simulink model "QAM_HF_Modell_Beispiel1"  (R2025b)
settings: Solver=VariableStepAuto  StartTime=0.0  StopTime=10.0  RelTol=1e-3
values from neighbouring files (symbols this model uses):
  ADC_delta = (ADC_Vmax - ADC_Vmin) / ADC_levels    (= 0.001953125)    [QAM_Bewertung_System_Parameter.m]
  alpha_LG = 0.001    [QAM_Bewertung_System_Parameter.m]
  c_init = complex(zeros(N_coef,1))    [QAM_Bewertung_System_Parameter.m]
  DAC_delta = (DAC_Vmax - DAC_Vmin) / DAC_levels    (= 0.000244140625)    [QAM_Bewertung_System_Parameter.m]
  freq_offset_Hz = 50    [QAM_Bewertung_System_Parameter.m]
  Fs = Rs * sps    (= 358400000)    [QAM_Bewertung_System_Parameter.m]
  Gain_DAC = V_dac_rms / sqrt(TX_Power)    [QAM_Bewertung_System_Parameter.m]
  Gain_rx_dB = 20*log10(Gain_rx_linear)    [QAM_Bewertung_System_Parameter.m]
  Gain_Tx_dB = 24    [QAM_Bewertung_System_Parameter.m]
  gainI_RX_dB = 0    [QAM_Bewertung_System_Parameter.m]
  gainI_TX_dB = 0.5    [QAM_Bewertung_System_Parameter.m]
  gainQ_RX_dB = 0.5    [QAM_Bewertung_System_Parameter.m]
  gainQ_TX_dB = 0.5    [QAM_Bewertung_System_Parameter.m]
  K_LG = 0.02    [QAM_Bewertung_System_Parameter.m]
  L_total_dB = FSPL_dB + L_gas_dB + L_rain_dB + L_sys_dB    [QAM_Bewertung_System_Parameter.m]
  LO_leakage_RX_dB = -30    [QAM_Bewertung_System_Parameter.m]
  LO_leakage_TX_dB = -35    [QAM_Bewertung_System_Parameter.m]
  M = 256    [QAM_Bewertung_System_Parameter.m]
  Memory = 1    [QAM_Bewertung_System_Parameter.m]
  mu = 5e-4    (= 0.0005)    [QAM_Bewertung_System_Parameter.m]
  mu_DPD = 1e-5    (= 1e-05)    [QAM_Bewertung_System_Parameter.m]
  numOrders = 3    [QAM_Bewertung_System_Parameter.m]
  P1dB_dBm = 20    [QAM_Bewertung_System_Parameter.m]
  P_TX_dBm = 10*log10(P_TX_W*1e3)    [QAM_Bewertung_System_Parameter.m]
  P_TX_W = 2    [QAM_Bewertung_System_Parameter.m]
  PAPR_dB = 6    [QAM_Bewertung_System_Parameter.m]
  phaseMismatch_RX_deg = 1    [QAM_Bewertung_System_Parameter.m]
  phaseMismatch_TX_deg = 1    [QAM_Bewertung_System_Parameter.m]
  PN_RX_std_deg = 0.01    [QAM_Bewertung_System_Parameter.m]
  PN_TX_std_deg = 0.01    [QAM_Bewertung_System_Parameter.m]
  R = 50    [QAM_Bewertung_System_Parameter.m]
  simulink_params = struct()    [QAM_Bewertung_System_Parameter.m]
  Z0 = 50    [QAM_Bewertung_System_Parameter.m]
libraries: dspstat3 x8, simulink_extras x4, dspmathops x3, simulink x2, commsink2 x2, commfilt2 x2, commdigbbndam3 x2, commrfcorlib x1, rfmathmodels2 x1, commrandsrc3 x1
settings Model: Creator=giand  LastModifiedBy=giand

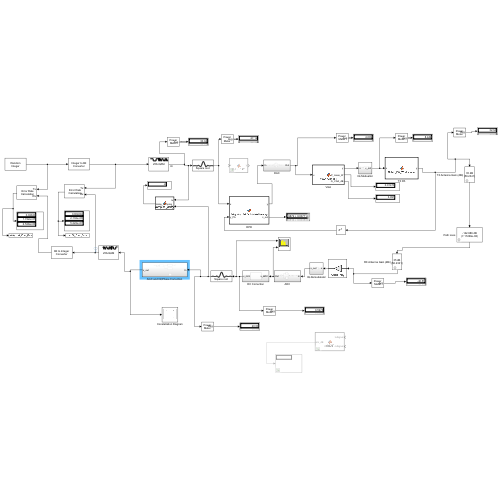
[thumbnail: Simulink's stored preview of the top-level diagram]
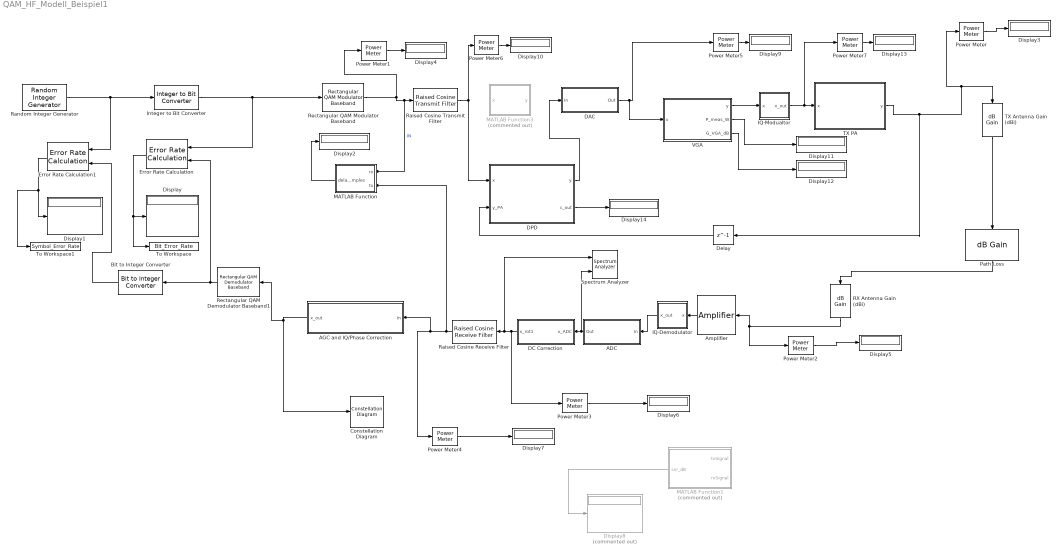
== system QAM_HF_Modell_Beispiel1 ==
  ADC : Subsystem
  AGC and IQ/Phase Correction : Subsystem
  Amplifier : rfmathmodels2/Amplifier  Model=cubic  Gain=Gain_rx_dB  Nonlinearity=OIP3  IIP3=Inf  OIP3=Inf  IP1dB=Inf  OP1dB=Inf  IPsat=Inf  OPsat=Inf  Table=[ -25, 5, -1; -10, 20, -2; 0, 27, 5; 5, 28, 12 ]  MagnitudeGainDB=0  Vsat=1  MagnitudeSmooth=2  PhaseGainRadian=-.45  PhaseSaturation=.88  PhaseSmooth=[ 3.43, 3.43 ]  InputScaleDB=0  AmAmParameters=[ 2.1587, 1.1517 ]  AmPmParameters=[ 4.0033, 9.1040 ]  OutputScaleDB=0  SimulateUsing=Interpreted execution  IncludeNoise=on  NoiseType=NF  NoiseTemperature=290  NF=NF_required_dB  NoiseFactor=2  SeedSource=auto  Seed=67987  SampleRate=1e6
  Bit to Integer Converter : simulink/Logic and Bit Operations/Bit to Integer Converter  nbits=k  bitOrder=MSB first  signedOutputValues=Unsigned  outDtype=Inherit via internal rule  outDtypeSigned=Inherit via internal rule
  Constellation Diagram : ConstellationDiagram  WindowPosition=[606.000000,-23.000000,853.000000,842.000000,]  Visible=on  ScopeFrameLocation=window
  DAC : Subsystem
  DC Correction : Subsystem
  DPD : MATLAB Function  TreatAsAtomicUnit=on
  Delay : Delay  DelayLength=1  InitialCondition=0
  Display{,1..7,9..14} (14 alike) : Display
  Display8 : Display  Commented=on
  Error Rate Calculation : commsink2/Error Rate Calculation  N=simulink_params.rrc_span*log2(M)  st_delay=0  cp_mode=Entire frame  subframe=[]  PMode=Port  WsName=ErrorVec  RsMode2=off  stop=off  numErr=100  maxBits=1e6
  Error Rate Calculation1 : commsink2/Error Rate Calculation  N=simulink_params.rrc_span  st_delay=0  cp_mode=Entire frame  subframe=[]  PMode=Port  WsName=ErrorVec  RsMode2=off  stop=off  numErr=100  maxBits=1e6
  IQ-Demodulator : Subsystem
  IQ-Modualtor : Subsystem
  Integer to Bit Converter : simulink/Logic and Bit Operations/Integer to Bit Converter  nbits=simulink_params.k  signedInputValues=Unsigned  bitOrder=MSB first  outDtype=Inherit via internal rule
      settings: LibrarySourceBlock=|
      | commutil2/Integer to Bit
      | Converter
  MATLAB Function : MATLAB Function  TreatAsAtomicUnit=on
  MATLAB Function1 : MATLAB Function  Commented=on  TreatAsAtomicUnit=on
  MATLAB Function3 : MATLAB Function  Commented=on  TreatAsAtomicUnit=on
  Path Loss : dspmathops/dB Gain  dB=-L_total_dB  intype=Amplitude
  Power Meter : dspstat3/Power Meter  Measurement=Average power  ReferenceLoad=R  OutputPowerUnits=dBm  WindowLength=256  OverlapLength=255  AllowArbitraryInputLength=off  ComputeCCDF=off  PowerRange=50  PowerResolution=0.1  CCDFOutput=Relative power (dB above average power)  ProbabilityVector=[ 10; 1; 0.1; 0.01; 0.001; 0.0001 ]  RelativePowerVector=[ 0; 3; 6; 9; 12 ]  ResetPort=off  SimulateUsing=Code generation
      settings: LibrarySourceBlock=commutil2/Power Meter
  Power Meter1 : dspstat3/Power Meter  Measurement=Average power  ReferenceLoad=1  OutputPowerUnits=dBm  WindowLength=256  OverlapLength=255  AllowArbitraryInputLength=on  ComputeCCDF=off  PowerRange=50  PowerResolution=0.1  CCDFOutput=Relative power (dB above average power)  ProbabilityVector=[ 10; 1; 0.1; 0.01; 0.001; 0.0001 ]  RelativePowerVector=[ 0; 3; 6; 9; 12 ]  ResetPort=off  SimulateUsing=Code generation
      settings: LibrarySourceBlock=commutil2/Power Meter
  Power Meter2 : dspstat3/Power Meter  Measurement=Average power  ReferenceLoad=R  OutputPowerUnits=dBm  WindowLength=256  OverlapLength=255  AllowArbitraryInputLength=off  ComputeCCDF=off  PowerRange=50  PowerResolution=0.1  CCDFOutput=Relative power (dB above average power)  ProbabilityVector=[ 10; 1; 0.1; 0.01; 0.001; 0.0001 ]  RelativePowerVector=[ 0; 3; 6; 9; 12 ]  ResetPort=off  SimulateUsing=Code generation
      settings: LibrarySourceBlock=commutil2/Power Meter
  Power Meter3 : dspstat3/Power Meter  Measurement=Average power  ReferenceLoad=R  OutputPowerUnits=dBm  WindowLength=256  OverlapLength=255  AllowArbitraryInputLength=off  ComputeCCDF=off  PowerRange=50  PowerResolution=0.1  CCDFOutput=Relative power (dB above average power)  ProbabilityVector=[ 10; 1; 0.1; 0.01; 0.001; 0.0001 ]  RelativePowerVector=[ 0; 3; 6; 9; 12 ]  ResetPort=off  SimulateUsing=Code generation
      settings: LibrarySourceBlock=commutil2/Power Meter
  Power Meter4 : dspstat3/Power Meter  Measurement=Average power  ReferenceLoad=1  OutputPowerUnits=dBm  WindowLength=256  OverlapLength=255  AllowArbitraryInputLength=off  ComputeCCDF=off  PowerRange=50  PowerResolution=0.1  CCDFOutput=Relative power (dB above average power)  ProbabilityVector=[ 10; 1; 0.1; 0.01; 0.001; 0.0001 ]  RelativePowerVector=[ 0; 3; 6; 9; 12 ]  ResetPort=off  SimulateUsing=Code generation
      settings: LibrarySourceBlock=commutil2/Power Meter
  Power Meter5 : dspstat3/Power Meter  Measurement=Average power  ReferenceLoad=R  OutputPowerUnits=dBm  WindowLength=256  OverlapLength=255  AllowArbitraryInputLength=on  ComputeCCDF=off  PowerRange=50  PowerResolution=0.1  CCDFOutput=Relative power (dB above average power)  ProbabilityVector=[ 10; 1; 0.1; 0.01; 0.001; 0.0001 ]  RelativePowerVector=[ 0; 3; 6; 9; 12 ]  ResetPort=off  SimulateUsing=Code generation
      settings: LibrarySourceBlock=commutil2/Power Meter
  Power Meter6 : dspstat3/Power Meter  Measurement=Average power  ReferenceLoad=1  OutputPowerUnits=dBm  WindowLength=256  OverlapLength=255  AllowArbitraryInputLength=on  ComputeCCDF=off  PowerRange=50  PowerResolution=0.1  CCDFOutput=Relative power (dB above average power)  ProbabilityVector=[ 10; 1; 0.1; 0.01; 0.001; 0.0001 ]  RelativePowerVector=[ 0; 3; 6; 9; 12 ]  ResetPort=off  SimulateUsing=Code generation
      settings: LibrarySourceBlock=commutil2/Power Meter
  Power Meter7 : dspstat3/Power Meter  Measurement=Average power  ReferenceLoad=R  OutputPowerUnits=dBm  WindowLength=256  OverlapLength=255  AllowArbitraryInputLength=on  ComputeCCDF=off  PowerRange=50  PowerResolution=0.1  CCDFOutput=Relative power (dB above average power)  ProbabilityVector=[ 10; 1; 0.1; 0.01; 0.001; 0.0001 ]  RelativePowerVector=[ 0; 3; 6; 9; 12 ]  ResetPort=off  SimulateUsing=Code generation
      settings: LibrarySourceBlock=commutil2/Power Meter
  RX Antenna Gain (dBi) : dspmathops/dB Gain  dB=G_TX_dBi  intype=Amplitude
  Raised Cosine Receive Filter : commfilt2/Raised Cosine Receive Filter  filtType=Square root  R=simulink_params.rrc_rolloff  filtSpan=simulink_params.rrc_span  N=simulink_params.sps  downFactor=simulink_params.sps  downOffset=0  filterGain=1  InputProcessing=Columns as channels (frame based)  RateOptions=Enforce single-rate processing  framing=Mute  checkCoeff=off  variableName=rcRxFilt  currentFiltSpan=10  D=5  inputOffset=0  sampMode=Mute  saveAsFlag=0  rateMode=Downsampling  checkGain=Normalized  launchFVT=on  roundingMode=Floor  overflowMode=off  coeffDataTypeStr=Inherit: Same word length as input  coeffMin=[]  coeffMax=[]  coeffLastDataTypeStr=Inherit: Same word length as input  accumDataTypeStr=Inherit: Same as product output  accumLastDataTypeStr=Inherit: Same as product output  outputDataTypeStr=Inherit: Same as accumulator  outputMin=[]  outputMax=[]  outputLastDataTypeStr=Inherit: Same as accumulator
  Raised Cosine Transmit Filter : commfilt2/Raised Cosine Transmit Filter  filtType=Square root  R=simulink_params.rrc_rolloff  filtSpan=simulink_params.rrc_span  N=simulink_params.sps  filterGain=1  InputProcessing=Columns as channels (frame based)  RateOptions=Enforce single-rate processing  framing=Mute  checkCoeff=off  variableName=rcTxFilt  checkGain=Normalized  sampMode=Mute  saveAsFlag=0  currentFiltSpan=10  D=(10)/2  launchFVT=on  roundingMode=Floor  overflowMode=off  coeffDataTypeStr=Inherit: Same word length as input  coeffMin=[]  coeffMax=[]  coeffLastDataTypeStr=Inherit: Same word length as input  outputDataTypeStr=Inherit: Same as accumulator  outputMin=[]  outputMax=[]  outputLastDataTypeStr=Inherit: Same as accumulator
  Random Integer Generator : commrandsrc3/Random Integer Generator  SetSize=simulink_params.M  SeedSource=Auto  Seed=0  SampleTime=1/simulink_params.Rs  SamplesPerFrame=simulink_params.spf  OutputDataType=double  SimulateUsing=Interpreted execution
  Rectangular QAM Demodulator Baseband1 : commdigbbndam3/Rectangular QAM Demodulator Baseband  M=M  OutType=Bit  DecType=Hard decision  VarSource=Dialog  Variance=1  Dec=Gray  Mapping=[0:15]  PowType=Average Power  MinDist=2  AvgPow=1  PeakPow=1  Ph=0  outDtype1=Inherit via internal rule  outDtype2=Inherit via internal rule  derotateFactorWordLen=16  derotateFactorDataTypeStr=Inherit: Same word length as input  derotateFactorLastDataTypeStr=Inherit: Same word length as input  denormFactorWordLen=16  denormFactorDataTypeStr=Inherit: Same word length as input  denormFactorLastDataTypeStr=Inherit: Same word length as input  prodOutWordLen=32  prodOutOverflowMode=Wrap  prodOutRoundingMode=Floor  prodOutOvFlMode=off  prodOutOvFlModeLastStrValue=off  sumWordLen=32
  Rectangular QAM Modulator Baseband : commdigbbndam3/Rectangular QAM Modulator Baseband  M=simulink_params.M  InType=Bit  Enc=Gray  Mapping=[0:15]  PowType=Average Power  MinDist=2  AvgPow=1  PeakPow=1  Ph=0  outDtype=double  outWordLen=16  outUDDataType=sfix(16)  outFracLenMode=Best precision  outFracLen=15  outDataTypeStr=double  outLastDataTypeStr=double
  Spectrum Analyzer : SpectrumAnalyzer  NumInputPorts=2  WindowPosition=[9.000000,57.000000,1520.000000,777.000000,]  Visible=on  ScopeFrameLocation=window  WindowInvariantSamplesPerUpdate=on  Span=358399999.99999994  StartFrequency=-179199999.99999997  StopFrequency=179199999.99999997  YLimits=[-47.4772 10.5436]
  TX Antenna Gain (dBi) : dspmathops/dB Gain  dB=G_TX_dBi  intype=Amplitude
  TX PA : MATLAB Function  TreatAsAtomicUnit=on
  To Workspace : ToWorkspace  VariableName=Bit_Error_Rate  SampleTime=-1
  To Workspace1 : ToWorkspace  VariableName=Symbol_Error_Rate  SampleTime=-1
  VGA : MATLAB Function  TreatAsAtomicUnit=on
  wires:
  Error Rate Calculation/1 -> Display/1, To Workspace/1
  Error Rate Calculation1/1 -> To Workspace1/1, Display1/1
  Random Integer Generator/1 -> Error Rate Calculation1/1, Integer to Bit Converter/1
  Integer to Bit Converter/1 -> Error Rate Calculation/1, Rectangular QAM Modulator Baseband/1
  Rectangular QAM Modulator Baseband/1 -> MATLAB Function/1(rx), Raised Cosine Transmit Filter/1, Power Meter1/1  "IN"
  Bit to Integer Converter/1 -> Error Rate Calculation1/2
  Rectangular QAM Demodulator Baseband1/1 -> Error Rate Calculation/2, Bit to Integer Converter/1
  MATLAB Function/1(delay_samples) -> Display2/1
  Path Loss/1 -> RX Antenna Gain (dBi)/1
  Power Meter1/1 -> Display4/1
  Power Meter/1 -> Display3/1
  TX Antenna Gain (dBi)/1 -> Path Loss/1
  RX Antenna Gain (dBi)/1 -> Power Meter2/1, Amplifier/1
  Power Meter2/1 -> Display5/1
  Power Meter3/1 -> Display6/1
  Power Meter4/1 -> Display7/1
  MATLAB Function1/1(snr_dB) -> Display8/1
  IQ-Demodulator/1(x_out) -> ADC/1(In)
  AGC and IQ/Phase Correction/1(x_out) -> Constellation Diagram/1, Rectangular QAM Demodulator Baseband1/1
  ADC/1(Out) -> Spectrum Analyzer/2, DC Correction/1(x_ADC)
  Amplifier/1 -> IQ-Demodulator/1(x)
  DC Correction/1(x_rot1) -> Power Meter3/1, Spectrum Analyzer/1, Raised Cosine Receive Filter/1
  Raised Cosine Receive Filter/1 -> MATLAB Function/2(tx), AGC and IQ/Phase Correction/1(In), Power Meter4/1
  Raised Cosine Transmit Filter/1 -> Power Meter6/1, DPD/1(x)
  Power Meter5/1 -> Display9/1
  Power Meter6/1 -> Display10/1
  VGA/1(y) -> IQ-Modualtor/1(x)
  VGA/2(P_meas_W) -> Display11/1
  VGA/3(G_VGA_dB) -> Display12/1
  IQ-Modualtor/1(x_out) -> Power Meter7/1, TX PA/1(x)
  TX PA/1(y) -> Delay/1, Power Meter/1, TX Antenna Gain (dBi)/1
  DAC/1(Out) -> VGA/1(x), Power Meter5/1
  Power Meter7/1 -> Display13/1
  DPD/1(y) -> DAC/1(In)
  DPD/2(c_out) -> Display14/1
  Delay/1 -> DPD/2(y_PA)

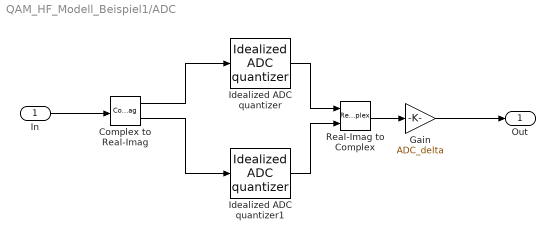
== system QAM_HF_Modell_Beispiel1/ADC ==
  In : Inport
  Complex to Real-Imag : ComplexToRealImag
  Gain : Gain  Gain=ADC_delta
  Idealized ADC quantizer : simulink_extras/Additional Discrete/Idealized ADC quantizer  NumberOfConverterBits=ADC_Bits  Vmin=ADC_Vmin  Vmax=ADC_Vmax  OutputDataType=double  OutputNegativeValues=on
  Idealized ADC quantizer1 : simulink_extras/Additional Discrete/Idealized ADC quantizer  NumberOfConverterBits=ADC_Bits  Vmin=ADC_Vmin  Vmax=ADC_Vmax  OutputDataType=double  OutputNegativeValues=on
  Real-Imag to Complex : RealImagToComplex
  Out : Outport  VectorParamsAs1DForOutWhenUnconnected=off
  wires:
  Idealized ADC quantizer/1 -> Real-Imag to Complex/1
  Idealized ADC quantizer1/1 -> Real-Imag to Complex/2
  Complex to Real-Imag/2 -> Idealized ADC quantizer1/1
  Gain/1 -> Out/1
  In/1 -> Complex to Real-Imag/1
  Complex to Real-Imag/1 -> Idealized ADC quantizer/1
  Real-Imag to Complex/1 -> Gain/1

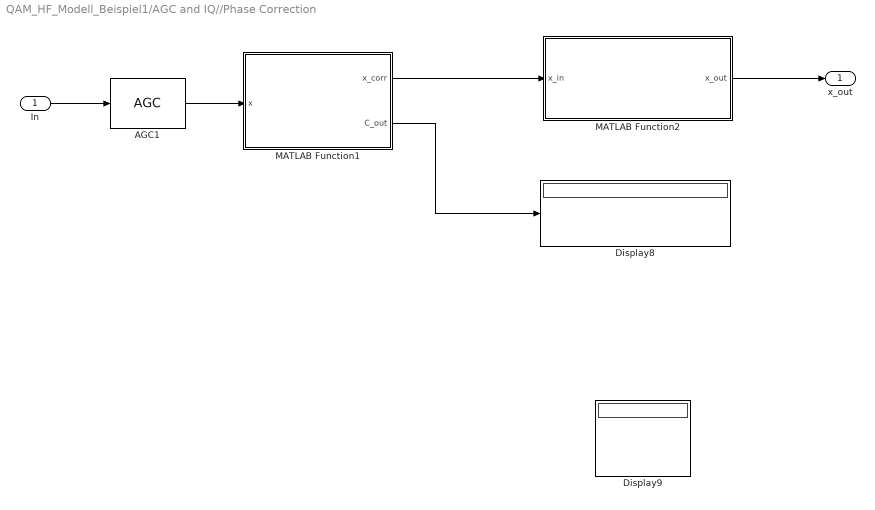
== system QAM_HF_Modell_Beispiel1/AGC and IQ//Phase Correction ==
  In : Inport
  AGC1 : commrfcorlib/AGC  LegacyMode=off  DetectorMethod=Rectifier  LoopMethod=Linear  UpdatePeriod=100  StepSize=0.1  AdaptationStepSize=0.001  DesiredOutputPower=1  AveragingLength=100  MaximumGain=30  MaxPowerGain=200  GainOutputPort=off  InputPowerOutputPort=off  SimulateUsing=Code generation
  Display8 : Display
  Display9 : Display
  MATLAB Function1 : MATLAB Function  TreatAsAtomicUnit=on
  MATLAB Function2 : MATLAB Function  TreatAsAtomicUnit=on
  x_out : Outport
  wires:
  MATLAB Function2/1(x_out) -> x_out/1
  MATLAB Function1/1(x_corr) -> MATLAB Function2/1(x_in)
  In/1 -> AGC1/1
  MATLAB Function1/2(C_out) -> Display8/1
  AGC1/1 -> MATLAB Function1/1(x)

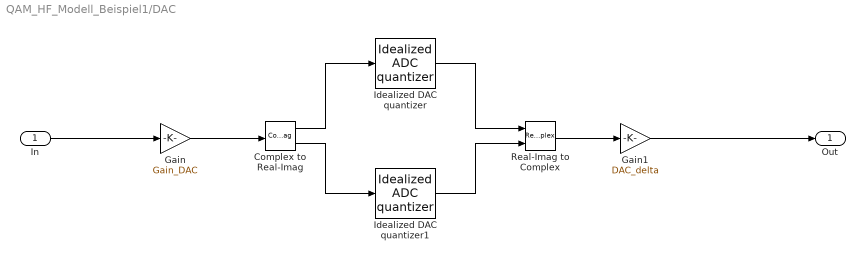
== system QAM_HF_Modell_Beispiel1/DAC ==
  In : Inport
  Complex to Real-Imag : ComplexToRealImag
  Gain : Gain  Gain=Gain_DAC
  Gain1 : Gain  Gain=DAC_delta
  Idealized DAC quantizer : simulink_extras/Additional Discrete/Idealized ADC quantizer  NumberOfConverterBits=DAC_Bits  Vmin=DAC_Vmin  Vmax=DAC_Vmax  OutputDataType=double  OutputNegativeValues=on
  Idealized DAC quantizer1 : simulink_extras/Additional Discrete/Idealized ADC quantizer  NumberOfConverterBits=DAC_Bits  Vmin=DAC_Vmin  Vmax=DAC_Vmax  OutputDataType=double  OutputNegativeValues=on
  Real-Imag to Complex : RealImagToComplex
  Out : Outport  VectorParamsAs1DForOutWhenUnconnected=off
  wires:
  Idealized DAC quantizer/1 -> Real-Imag to Complex/1
  Idealized DAC quantizer1/1 -> Real-Imag to Complex/2
  Complex to Real-Imag/2 -> Idealized DAC quantizer1/1
  In/1 -> Gain/1
  Complex to Real-Imag/1 -> Idealized DAC quantizer/1
  Real-Imag to Complex/1 -> Gain1/1
  Gain/1 -> Complex to Real-Imag/1
  Gain1/1 -> Out/1

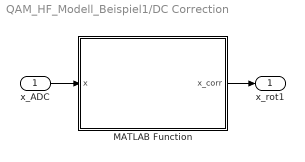
== system QAM_HF_Modell_Beispiel1/DC Correction ==
  x_ADC : Inport
  MATLAB Function : MATLAB Function  TreatAsAtomicUnit=on
  x_rot1 : Outport
  wires:
  x_ADC/1 -> MATLAB Function/1(x)
  MATLAB Function/1(x_corr) -> x_rot1/1

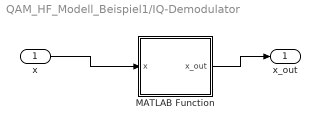
== system QAM_HF_Modell_Beispiel1/IQ-Demodulator ==
  x : Inport
  MATLAB Function : MATLAB Function  TreatAsAtomicUnit=on
  x_out : Outport
  wires:
  x/1 -> MATLAB Function/1(x)
  MATLAB Function/1(x_out) -> x_out/1

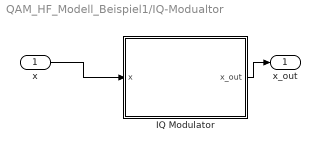
== system QAM_HF_Modell_Beispiel1/IQ-Modualtor ==
  x : Inport
  IQ Modulator : MATLAB Function  TreatAsAtomicUnit=on
  x_out : Outport
  wires:
  x/1 -> IQ Modulator/1(x)
  IQ Modulator/1(x_out) -> x_out/1

== matlab function QAM_HF_Modell_Beispiel1/VGA ==
  data: x input; R parameter; Gain_Tx_dB parameter; P_TX_W parameter; K_LG parameter; y output; P_meas_W output; G_VGA_dB output; alpha_LG parameter
function [y,P_meas_W,G_VGA_dB] = VGA_Control(x,R,Gain_Tx_dB,P_TX_W,K_LG,alpha_LG)

% Persistent states
persistent G_dB_internal Pavg

if isempty(G_dB_internal)
    G_dB_internal = 5;      % initial VGA gain
    Pavg = 0;
end

% Constants
coupler_dB = -20;

% Convert gains
G_amp = 10^(G_dB_internal/20);
PA_gain_amp = 10^(Gain_Tx_dB/20);
coupler_amp = 10^(coupler_dB/20);

% Apply VGA
y = G_amp .* x;

% PA output signal
x_pa = PA_gain_amp .* y;

% Coupler signal
x_cpl = coupler_amp .* x_pa;

% Instantaneous power (FRAME POWER)
P_inst = mean(abs(x_cpl).^2) / R;

% Exponential moving average (Power detector)
Pavg = (1 - alpha_LG) * Pavg + alpha_LG * P_inst;

P_meas_W = Pavg;

% Target power at coupler
P_target_meas = P_TX_W * 10^(coupler_dB/10);

% Control error
err = P_target_meas - P_meas_W;

% Gain update (scaled to dB domain)
G_dB_internal = G_dB_internal + K_LG * err * 50;

% VGA limits
if G_dB_internal > 20
    G_dB_internal = 20;
end

if G_dB_internal < -10
    G_dB_internal = -10;
end

% Output gain
G_VGA_dB = G_dB_internal;

end

== matlab function QAM_HF_Modell_Beispiel1/DPD ==
  data: x input double; y_PA input double; y output double; c_init parameter double; mu_DPD parameter; Memory parameter; c_out output double; numOrders parameter
function [y, c_out] = Adaptive_DPD_StableMemory(x, y_PA, c_init, mu_DPD, Memory, numOrders)
% Adaptive DPD für PA mit Cubic + Memory-Term
%
% Inputs:
%   x         : Input Signal (vor PA, complex double)
%   y_PA      : PA Output Signal als Feedback (complex double)
%   c_init    : Initiale Koeffizienten [N_coef x 1], complex
%   mu_DPD    : Schrittweite NLMS
%   Memory    : Anzahl Memory-Taps (0 = nur instantan)
%   numOrders : Polynom-Ordnung (z.B. 3)
%
% Outputs:
%   y      : Predistortiertes Signal
%   c_out  : Aktuelle Koeffizienten nach Update

x = complex(x(:));
y_PA = complex(y_PA(:));
N = length(x);
N_coef = numOrders*(Memory+1);

% Initialisierung
c = complex(c_init(:));
y = complex(zeros(N,1));
c_out = c;

% Feedback Delay 1 Sample
y_PA_delayed = [0; y_PA(1:end-1)];

% Sample-by-Sample NLMS
for n = 1:N
    % Regressor u bauen (Memory + Polynom)
    u = complex(zeros(N_coef,1));
    idx = 1;
    for m = 0:Memory
        for p = 1:numOrders
            if n-m > 0
                u(idx) = x(n-m) * abs(x(n-m))^(p-1);
            else
                u(idx) = 0;
            end
            idx = idx + 1;
        end
    end
    
    % Predistortion anwenden
    y(n) = c' * u;
    
    % Fehler berechnen
    e = y_PA_delayed(n) - y(n);
    
    % NLMS Update (normierter LMS)
    norm_u = max(sum(abs(u).^2), 1e-12);
    c = c + mu_DPD * conj(e) * u / norm_u;
end

c_out = c;

end

== matlab function QAM_HF_Modell_Beispiel1/IQ-Modualtor/IQ Modulator ==
  data: x input; x_out output; gainI_TX_dB parameter; gainQ_TX_dB parameter; phaseMismatch_TX_deg parameter; LO_leakage_TX_dB parameter; PN_TX_std_deg parameter; freq_offset_Hz parameter; Fs parameter
function x_out = IQ_Modulator_Block(x, gainI_TX_dB, gainQ_TX_dB, ...
phaseMismatch_TX_deg, LO_leakage_TX_dB, PN_TX_std_deg, ...
freq_offset_Hz, Fs)

N = length(x);

%% 1. Real / Imag
I = real(x);
Q = imag(x);

%% 2. Gain & Phase Mismatch
gI = 10^(gainI_TX_dB/20);
gQ = 10^(gainQ_TX_dB/20);
phi = deg2rad(phaseMismatch_TX_deg);

I_new = gI*I*cos(phi) - gQ*Q*sin(phi);
Q_new = gI*I*sin(phi) + gQ*Q*cos(phi);

%% 3. LO Leakage
LO_leakage = 10^(LO_leakage_TX_dB/20);
I_new = I_new + LO_leakage;
Q_new = Q_new + LO_leakage;

x_complex = I_new + 1j*Q_new;

%% 4. Phase Noise
phi_PN = deg2rad(PN_TX_std_deg) * randn(N,1);

%% 5. Frequency Offset
n = (0:N-1)';
phi_freq = 2*pi*freq_offset_Hz/Fs * n;

%% 6. Total Phase Rotation
x_out = x_complex .* exp(1j*(phi_PN + phi_freq));

end

== matlab function QAM_HF_Modell_Beispiel1/AGC and IQ//Phase Correction/MATLAB Function2 ==
  data: x_in input; x_out output; M parameter; PN_TX_std_deg parameter; PN_RX_std_deg parameter
function x_out = EKF_Phase_Tracking_Stable(x_in,M,PN_TX_std_deg,PN_RX_std_deg)

persistent phi_est freq_est P levels Q R_base

N = length(x_in);
x_out = complex(zeros(N,1));

sigma_phi = deg2rad(sqrt(PN_TX_std_deg^2 + PN_RX_std_deg^2));

%% QAM Levels
if isempty(levels)
    sqrtM = sqrt(M);
    levels = -(sqrtM-1):2:(sqrtM-1);
    levels = levels ./ sqrt(mean(levels.^2)*2);
end

%% EKF Initialization
if isempty(phi_est), phi_est = 0; end
if isempty(freq_est), freq_est = 0; end
if isempty(P), P = eye(2)*1e-3; end
if isempty(Q), Q = diag([sigma_phi^2 (sigma_phi/50)^2]); end
if isempty(R_base), R_base = (sigma_phi/2)^2; end

for n=1:N

    %% Prediction
    x_pred = [phi_est + freq_est ; freq_est];

    F = [1 1;0 1];
    P = F*P*F' + Q;

    %% Phase correction
    x_corr = x_in(n)*exp(-1j*x_pred(1));

    %% Decision Directed Symbol
    [~,ir] = min(abs(real(x_corr)-levels));
    [~,ii] = min(abs(imag(x_corr)-levels));
    s_hat = levels(ir) + 1j*levels(ii);

    %% Phase detector
    z = angle(x_corr*conj(s_hat));

    %% Adaptive measurement noise
    R = max(R_base, z^2);

    %% Measurement matrix
    H = [1 0];

    %% Kalman gain
    S = H*P*H' + R;
    K = P*H'/S;

    %% Update
    x_upd = x_pred + K*(z - H*x_pred);

    % Joseph stabilized covariance update
    I = eye(2);
    P = (I-K*H)*P*(I-K*H)' + K*R*K';

    phi_est  = x_upd(1);
    freq_est = x_upd(2);

    %% Phase wrap (sehr wichtig für lange Simulationen)
    phi_est = mod(phi_est + pi, 2*pi) - pi;

    %% Output
    x_out(n) = x_in(n)*exp(-1j*phi_est);

end

end

== matlab function QAM_HF_Modell_Beispiel1/MATLAB Function1 ==
  data: txSignal input; rxSignal input; snr_dB output
function snr_dB = calcSNR(txSignal, rxSignal)
% calcSNR - Berechnet das Signal-Rausch-Verhältnis in dB
%
% Eingänge:
%   rxSignal - empfangenes Signal nach AGC/Filter
%   txSignal - ursprüngliches Sendesignal (Referenz)
%
% Ausgang:
%   snr_dB  - SNR in Dezibel

    % Noise berechnen
    noise = rxSignal - txSignal;

    % Leistung von Signal und Noise
    P_signal = mean(abs(txSignal).^2);
    P_noise  = mean(abs(noise).^2);

    % SNR in dB
    snr_dB = 10 * log10(P_signal / P_noise);
end

== matlab function QAM_HF_Modell_Beispiel1/MATLAB Function ==
  data: rx input; delay_samples output; tx input
function delay_samples = compute_delay(rx, tx)
    [xc, lags] = xcorr(rx, tx);
    [~, idx] = max(abs(xc));
    delay_samples = lags(idx);
end

== matlab function QAM_HF_Modell_Beispiel1/IQ-Demodulator/MATLAB Function ==
  data: x input; x_out output; gainI_RX_dB parameter; gainQ_RX_dB parameter; phaseMismatch_RX_deg parameter; LO_leakage_RX_dB parameter; PN_RX_std_deg parameter; freq_offset_Hz parameter; Fs parameter
function x_out = IQ_Demodulator_Block(x, gainI_RX_dB, gainQ_RX_dB, ...
phaseMismatch_RX_deg, LO_leakage_RX_dB, PN_RX_std_deg, ...
freq_offset_Hz, Fs)

N = length(x);

%% 1. Real / Imag
I = real(x);
Q = imag(x);

%% 2. Gain & Phase Mismatch
gI = 10^(gainI_RX_dB/20);
gQ = 10^(gainQ_RX_dB/20);
phi = deg2rad(phaseMismatch_RX_deg);

I_new = gI*I*cos(phi) - gQ*Q*sin(phi);
Q_new = gI*I*sin(phi) + gQ*Q*cos(phi);

%% 3. LO Leakage
LO_leakage = 10^(LO_leakage_RX_dB/20);
I_new = I_new + LO_leakage;
Q_new = Q_new + LO_leakage;

x_complex = I_new + 1j*Q_new;

%% 4. Phase Noise
phi_PN = deg2rad(PN_RX_std_deg) * randn(N,1);

%% 5. Frequency Offset
n = (0:N-1)';
phi_freq = 2*pi*freq_offset_Hz/Fs * n;

%% 6. Total Rotation
x_out = x_complex .* exp(1j*(phi_PN + phi_freq));

end

== matlab function QAM_HF_Modell_Beispiel1/DC Correction/MATLAB Function ==
  data: x input; x_corr output; alpha parameter
function x_corr = DC_Offset_Removal(x, alpha)

persistent dc_I dc_Q

if isempty(dc_I)
    dc_I = 0;
    dc_Q = 0;
end

N = length(x);
x_corr = complex(zeros(N,1));

for n = 1:N
    
    I = real(x(n));
    Q = imag(x(n));
    
    % Running mean
    dc_I = (1-alpha)*dc_I + alpha*I;
    dc_Q = (1-alpha)*dc_Q + alpha*Q;
    
    % Removal
    x_corr(n) = complex(I - dc_I, Q - dc_Q);

end

end

== matlab function QAM_HF_Modell_Beispiel1/AGC and IQ//Phase Correction/MATLAB Function1 ==
  data: x input; x_corr output; mu parameter; M parameter; C_out output
function [x_corr, C_out] = IQ_Imbalance_Correction(x, mu, M)
% Adaptive IQ Imbalance Correction (NLMS Version)
% Optimiert für Simulink / Streaming Receiver

persistent C constellation

N = length(x);
x_corr = complex(zeros(N,1));

%% Initialisierung
if isempty(C)
    C = eye(2);
end

if isempty(constellation)
    constellation = qammod(0:M-1, M, 'UnitAveragePower', true).';
end

eps_norm = 1e-6;

%% Hauptloop
for n = 1:N

    % Eingangssignal
    IQ_vec = [real(x(n)); imag(x(n))];

    % Korrekturmatrix anwenden
    IQ_corr = C * IQ_vec;

    x_corr(n) = complex(IQ_corr(1), IQ_corr(2));

    %% Decision Directed Reference
    [~, idx] = min(abs(x_corr(n) - constellation));
    s_ref = constellation(idx);

    ref_vec = [real(s_ref); imag(s_ref)];

    %% Fehlervektor
    e = ref_vec - IQ_corr;

    %% Normalized LMS
    norm_factor = eps_norm + (IQ_vec.' * IQ_vec);

    mu_eff = mu / norm_factor;

    %% Update
    C = C + mu_eff * (e * IQ_vec.');

end

C_out = C;

end

== matlab function QAM_HF_Modell_Beispiel1/TX PA ==
  data: x input; P_TX_dBm parameter; y output; Gain_Tx_dB parameter; P1dB_dBm parameter; Z0 parameter; PAPR_dB parameter
function y = Cubic_PA_Workspace(x, P_TX_dBm, Gain_Tx_dB, P1dB_dBm, Z0, PAPR_dB)

%% Peakleistung
P_peak_dBm = P_TX_dBm + PAPR_dB;
P_peak_W   = 10^(P_peak_dBm/10)/1000;

%% Linear Gain
a1 = 10^(Gain_Tx_dB/20);

%% 1dB Compression
P1dB_W = 10^(P1dB_dBm/10)/1000;
A_1dB  = sqrt(P1dB_W*Z0);

%% Cubic coefficient
a3 = a1*(10^(-1/20)-1)/A_1dB^2;

%% Memory coefficient (klein!)
b3 = 0.1*a3;

%% Delay
x_delay = [0; x(1:end-1)];

%% PA Modell
y = a1*x ...
  + a3*abs(x).^2 .* x ...
  + b3*abs(x_delay).^2 .* x;

%% Backoff Warnung
Backoff_dB = P1dB_dBm - P_peak_dBm;

if Backoff_dB < 0
    warning('Peak liegt über P1dB! Nichtlinearität unvermeidbar.');
end

end

== matlab function QAM_HF_Modell_Beispiel1/MATLAB Function3 ==
  data: x input; y output; Gain_Tx_dB parameter; P1dB_dBm parameter; Z0 parameter
function y = Static_DPD(x, Gain_Tx_dB, P1dB_dBm, Z0)

% Static Digital Predistortion
% kompensiert Cubic-PA Nichtlinearität

%% Linear Gain des PA
a1 = 10^(Gain_Tx_dB/20);

%% Spannung bei 1 dB Compression
P1dB_W = 10^(P1dB_dBm/10)/1000;
A_1dB  = sqrt(P1dB_W*Z0);

%% Cubic Koeffizient des PA
a3 = a1*(10^(-1/20)-1)/A_1dB^2;

%% DPD Koeffizienten
b1 = 1;                     % Gain unverändert (VGA übernimmt Level)
b3 = -a3/(a1^3);            % Cubic Inversion

%% Predistortion
y = b1*x + b3*abs(x).^2 .* x;

end
